simulink model "funcion_2"  (R2019a)
settings: Solver=VariableStepAuto  StartTime=0.0  StopTime=10.0  RelTol=1e-3
values from neighbouring files (symbols this model uses):
  a = -2.0000e-01    (= -0.2)    [programa_nodos.m]
  b = -1.6000e-02    (= -0.016)    [programa_nodos.m]
  c = -6.4000e-04    (= -0.00064)    [programa_nodos.m]
  d = -1.2800e-05    (= -1.28e-05)    [programa_nodos.m]
  h = 1.0000e+00    (= 1)    [programa_nodos.m]
  hdis = hdis'    [programa_nodos.m]
  i = 1.0000e+00    (= 1)    [programa_nodos.m]
  j = 1.0000e+00    (= 1)    [programa_nodos.m]
  k = -2.5000e-01    (= -0.25)    [programa_nodos.m]
  l = -3.3141e+00    (= -3.3141)    [programa_nodos.m]
  m = -4.3146e+00    (= -4.3146)    [programa_nodos.m]
  n = 1.0000e+00    (= 1)    [programa_nodos.m]
  o = 1.0000e+00    (= 1)    [programa_nodos.m]
  s = 1.3156e+02    (= 131.56)    [programa_nodos.m]
  tm = 0.5    [programa_nodos.m]
  v = 1.2563e+00    (= 1.2563)    [programa_nodos.m]
  z0 = 0.5    [programa_nodos.m]
  z1 = 0.00000001    (= 1e-08)    [programa_nodos.m]
  z2 = 0.00000001    (= 1e-08)    [programa_nodos.m]
  z3 = 0.00000001    (= 1e-08)    [programa_nodos.m]
  z4 = 0.00000001    (= 1e-08)    [programa_nodos.m]
  z5 = 0.00000001    (= 1e-08)    [programa_nodos.m]
  z6 = 0.00000001    (= 1e-08)    [programa_nodos.m]
  z7 = 0.00000001    (= 1e-08)    [programa_nodos.m]
undefined symbols (not defined in the file or in its folder): A2, adis, B2, bdis, C2, cdis, g, u1, u2, u3, u4, u5, u6, u7, u8, u9
libraries: simulink x1
settings Model: Creator=Alejoxbg  LastModifiedBy=Alejoxbg

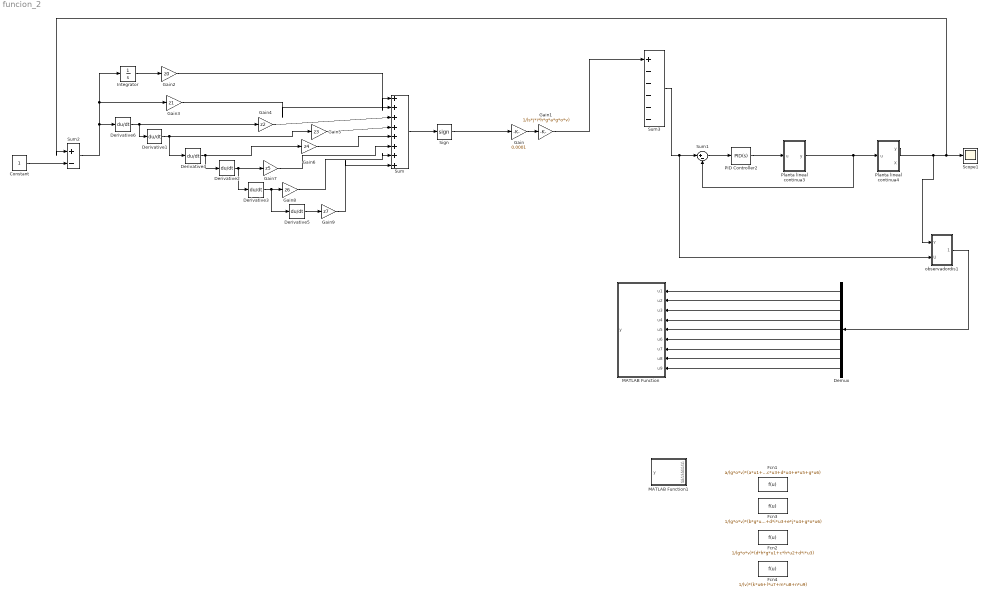
== system funcion_2 ==
  Constant : Constant
  Demux : Demux  Outputs=9
  Derivative{1..6} (6 alike) : Derivative
  Fcn1 : Fcn  Expr=a/(g*o*v)*(a*u1+b*u2+c*u3+d*u4+e*u5+g*u6)
  Fcn2 : Fcn  Expr=1/(g*o*v)*(d*h*g*u1+c*h*u2+d*i*u3)
  Fcn3 : Fcn  Expr=1/(g*o*v)*(b*g*u1+c*h*u2+d*i*u3+e*j*u4+g*o*u6)
  Fcn4 : Fcn  Expr=1/(v)*(k*u6+l*u7+m*u8+n*u9)
  Gain : Gain  Gain=0.0001
  Gain1 : Gain  Gain=1/(s*j*i*h*g*a*g*o*v)
  Gain2 : Gain  Gain=z0
  Gain3 : Gain  Gain=z1
  Gain4 : Gain  Gain=z2
  Gain5 : Gain  Gain=z3
  Gain6 : Gain  Gain=z4
  Gain7 : Gain  Gain=z5
  Gain8 : Gain  Gain=z6
  Gain9 : Gain  Gain=z7
  Integrator : Integrator
  MATLAB Function : MATLAB Function  TreatAsAtomicUnit=on
  MATLAB Function1 : MATLAB Function  TreatAsAtomicUnit=on
  PID Controller2 : simulink/Continuous/PID Controller  Controller=PID  Form=Parallel  TimeDomain=Continuous-time  SampleTime=-1  IntegratorMethod=Forward Euler  FilterMethod=Forward Euler  ControllerParametersSource=internal  P=12.1148539818802  I=1.25631014904339  D=27.6845650272969  UseFilter=on  N=4.3146205312046  TunerSelectOption=Transfer Function Based (PID Tuner App)  InitialConditionSource=internal  InitialConditionForIntegrator=0  InitialConditionForFilter=0  DifferentiatorICPrevScaledInput=0  ExternalReset=none  TrackingMode=off  Kt=1  LimitOutput=off  UpperSaturationLimit=inf  LowerSaturationLimit=-inf  LinearizeAsGain=on  AntiWindupMode=none  Kb=1  POutMin=[]  POutMax=[]  IOutMin=[]  IOutMax=[]  DOutMin=[]  DOutMax=[]  NOutMin=[]  NOutMax=[]  SumOutMin=[]  SumOutMax=[]  SaturationOutMin=[]  SaturationOutMax=[]  PParamMin=[]  PParamMax=[]  IParamMin=[]  IParamMax=[]  DParamMin=[]  DParamMax=[]  NParamMin=[]  NParamMax=[]  KbParamMin=[]  KbParamMax=[]  KtParamMin=[]  KtParamMax=[]  KbOutMin=[]  KbOutMax=[]  KtOutMin=[]  KtOutMax=[]  IntegratorOutMin=[]  IntegratorOutMax=[]  FilterOutMin=[]  FilterOutMax=[]  SumI1OutMin=[]  SumI1OutMax=[]  SumI2OutMin=[]  SumI2OutMax=[]  SumI3OutMin=[]  SumI3OutMax=[]  SumI4OutMin=[]  SumI4OutMax=[]  SumDOutMin=[]  SumDOutMax=[]  DifferentiatorOutMin=[]  DifferentiatorOutMax=[]  FilterDiffOutCoefMin=[]  FilterDiffOutCoefMax=[]  ReciprocalOutMin=[]  ReciprocalOutMax=[]  SumDenOutMin=[]  SumDenOutMax=[]  SumNumOutMin=[]  SumNumOutMax=[]  DivideOutMin=[]  DivideOutMax=[]  IntegratorContinuousStateAttributes=''  IntegratorStateMustResolveToSignalObject=off  IntegratorRTWStateStorageClass=Auto  FilterContinuousStateAttributes=''  FilterStateMustResolveToSignalObject=off  FilterRTWStateStorageClass=Auto  ParallelPVariant=InternalParameters  IdealPVariant=Disabled  IVariant=InternalParameters  DVariant=InternalParameters  IntegratorVariant=Continuous  SatVariant=Disabled  AWVariant=Passthrough  PCopyVariant=Disabled  TRVariant=Disabled  FdbkBlocksVariant=Forward  IdealPFdbkVariant=Disabled  SatFdbkVariant=Disabled  DerivativeFilterVariant=ContFilter  NVariant=InternalParameters  NCopyVariant=Disabled  FilterICVariant=InternalICsFilter  IntegratorICVariant=InternalICs  ExternalResetVariant=Disabled  TRSumVariant=Passthrough  SumFdbkVariant=Disabled  SumVariant=Sum_PID
  Planta lineal continua3 : Subsystem
  Planta lineal continua4 : Subsystem
  Scope1 : Scope
  Sign : Signum  ZeroCross=off
  Sum : Sum  Inputs=|++++++++
  Sum1 : Sum  Inputs=|+-
  Sum2 : Sum  Inputs=|+-
  Sum3 : Sum  Inputs=|+-----
  observadordis1 : Subsystem
  wires:
  Planta lineal continua3/1(y) -> Planta lineal continua4/1(u), Sum1/2
  Sum1/1 -> PID Controller2/1
  Constant/1 -> Sum2/2
  observadordis1/1(xgorro) -> Demux/1
  PID Controller2/1 -> Planta lineal continua3/1(u)
  Planta lineal continua4/1(y) -> Sum2/1, Scope1/1, observadordis1/1(Y)
  Sum2/1 -> Derivative6/1, Gain3/1, Integrator/1
  Gain/1 -> Gain1/1
  Integrator/1 -> Gain2/1
  Sum/1 -> Sign/1
  Sign/1 -> Gain/1
  Gain2/1 -> Sum/1
  Gain3/1 -> Sum/2
  Gain4/1 -> Sum/3
  Derivative6/1 -> Derivative1/1, Gain4/1
  Gain5/1 -> Sum/4
  Derivative1/1 -> Derivative4/1, Gain5/1
  Derivative4/1 -> Derivative2/1, Gain6/1
  Gain6/1 -> Sum/5
  Derivative2/1 -> Derivative3/1, Gain7/1
  Gain7/1 -> Sum/6
  Derivative3/1 -> Derivative5/1, Gain8/1
  Gain8/1 -> Sum/7
  Derivative5/1 -> Gain9/1
  Gain9/1 -> Sum/8
  Gain1/1 -> Sum3/1
  Sum3/1 -> observadordis1/2(U), Sum1/1
  Demux/1 -> MATLAB Function/1(u1)
  Demux/2 -> MATLAB Function/2(u2)
  Demux/3 -> MATLAB Function/3(u3)
  Demux/4 -> MATLAB Function/4(u4)
  Demux/5 -> MATLAB Function/5(u5)
  Demux/6 -> MATLAB Function/6(u6)
  Demux/7 -> MATLAB Function/7(u7)
  Demux/8 -> MATLAB Function/8(u8)
  Demux/9 -> MATLAB Function/9(u9)

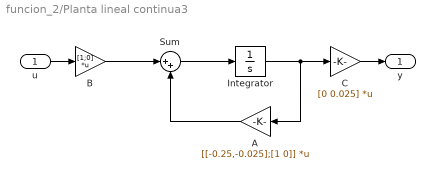
== system funcion_2/Planta lineal continua3 ==
  u : Inport
  A : Gain  Gain=[[-0.25,-0.025];[1 0]]  Multiplication=Matrix(K*u) (u vector)
  B : Gain  Gain=[1;0]  Multiplication=Matrix(K*u) (u vector)
  C : Gain  Gain=[0 0.025]  Multiplication=Matrix(K*u) (u vector)
  Integrator : Integrator
  Sum : Sum  Inputs=|++
  y : Outport
  wires:
  C/1 -> y/1
  u/1 -> B/1
  Integrator/1 -> A/1, C/1
  A/1 -> Sum/2
  Sum/1 -> Integrator/1
  B/1 -> Sum/1

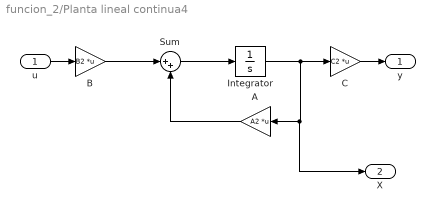
== system funcion_2/Planta lineal continua4 ==
  u : Inport
  A : Gain  Gain=A2  Multiplication=Matrix(K*u) (u vector)
  B : Gain  Gain=B2  Multiplication=Matrix(K*u) (u vector)
  C : Gain  Gain=C2  Multiplication=Matrix(K*u) (u vector)
  Integrator : Integrator
  Sum : Sum  Inputs=|++
  y : Outport
  X : Outport  Port=2
  wires:
  C/1 -> y/1
  u/1 -> B/1
  Integrator/1 -> X/1, A/1, C/1
  A/1 -> Sum/2
  Sum/1 -> Integrator/1
  B/1 -> Sum/1

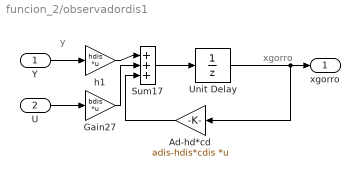
== system funcion_2/observadordis1 ==
  note: xgorro
  note: y
  Y : Inport
  U : Inport  Port=2
  Ad-hd*cd : Gain  Gain=adis-hdis*cdis  Multiplication=Matrix(K*u) (u vector)  SampleTime=tm
  Gain27 : Gain  Gain=bdis  Multiplication=Matrix(K*u) (u vector)  SampleTime=tm
  Sum17 : Sum  Inputs=|+++
  Unit Delay : UnitDelay  SampleTime=tm  HasFrameUpgradeWarning=on
  h1 : Gain  Gain=hdis  Multiplication=Matrix(K*u) (u vector)  SampleTime=tm
  xgorro : Outport
  wires:
  Sum17/1 -> Unit Delay/1
  h1/1 -> Sum17/1
  Unit Delay/1 -> Ad-hd*cd/1, xgorro/1
  Ad-hd*cd/1 -> Sum17/3
  Gain27/1 -> Sum17/2
  Y/1 -> h1/1
  U/1 -> Gain27/1

== matlab function funcion_2/MATLAB Function1 ==
  data: u1 input; y output; u2 input; u3 input; u4 input; u5 input; u6 input; u7 input; u8 input; u9 input
function y = fcn(u1,u2,u3,u4,u5,u6,u7,u8,u9)
a=1.1520e-07
 b=-2.0000e-01
 c=-1.6000e-02  
 d=-6.4000e-04  
 e=-1.2800e-05  
 f=-1.0240e-07 
 g=2.5000e-02
 h=1.0000e+00
 i=1.0000e+00
 j=1.0000e+00
 k=1.0000e+00
 l=-2.5000e-01
 m=-3.3141e+00
 n=-4.3146e+00
 o=1.0000e+00
 p=1.0000e+00
 q=-2.9862e+00
 r=-4.3146e+00
 s=-3.1408e-02
 t=1.3156e+02
 u=1.1945e+02
 v=1.2563e+00
y = a/(g*o*v)*(a*u1+b*u2+c*u3+d*u4+e*u5+g*u6);

== matlab function funcion_2/MATLAB Function ==
  data: u1 input; y output; u2 input; u3 input; u4 input; u5 input; u6 input; u7 input; u8 input; u9 input
function y = fcn(u1,u2,u3,u4,u5,u6,u7,u8,u9)
  a=1.1520e-07
 b=-2.0000e-01
 c=-1.6000e-02  
 d=-6.4000e-04  
 e=-1.2800e-05  
 f=-1.0240e-07 
 g=2.5000e-02
 h=1.0000e+00
 i=1.0000e+00
 j=1.0000e+00
 k=1.0000e+00
 l=-2.5000e-01
 m=-3.3141e+00
 n=-4.3146e+00
 o=1.0000e+00
 p=1.0000e+00
 q=-2.9862e+00
 r=-4.3146e+00
 s=-3.1408e-02
 t=1.3156e+02
 u=1.1945e+02
 v=1.2563e+00
y = s*j*i*h*g*a*a*(a*u1+b*u2+c*u3+d*u4+e*u5+g*u7)+s*j*i*h*g*a*(b*g*u1+c*h*u2+d*i*u3+e*j*u4+g*o*u6)+s*j*i*h*g*a*(d*h*g*u1+d*h*u2+d*i*u3)+s*j*i*h*g*a*g*o(k*u6+l*u7+m*u8+n*u9)+s*j*i*h*g*a*g*o*v*u;
